simulink subsystem "rss_CurrCtlHybr"  (R2023a)
settings: Solver=VariableStepAuto  StartTime=0.0  StopTime=10.0  RelTol=1e-3
undefined symbols (not defined in the file): bit, Cdbl_indPhIndcMaxVal, Cdbl_indPhIndcPeakVal, Cdbl_iPhCurrMaxVal, Cdbl_iPhCurrPeakVal, Cdbl_nElecAgSpdMaxVal, Cdbl_nElecAgSpdPeakVal, Cdbl_psiPermMagFlxMaxVal, Cdbl_psiPermMagFlxPeakVal, Cdbl_uPhVltgMaxVal, Cdbl_uSplyVltgPeakVal, dt_Standardize_s16p15b0, ENM_MOTO_STATUS, Gbol_flgDaxQaxCurrClpFlg_C, Gu16_indDaxIndc_C, Gu16_indQaxIndc_C, Gu16_psiPermMagFlx_C
libraries: lib_conversion x18, lib_configurable_parameter x6, lib_discrete_time_PI_controller32bit x2, simulink x1
settings Model: Creator=CAV2OFO  LastModifiedBy=xiaoqiang.yuan
settings OptimizationCC: ReuseModelBlockBuffer=off

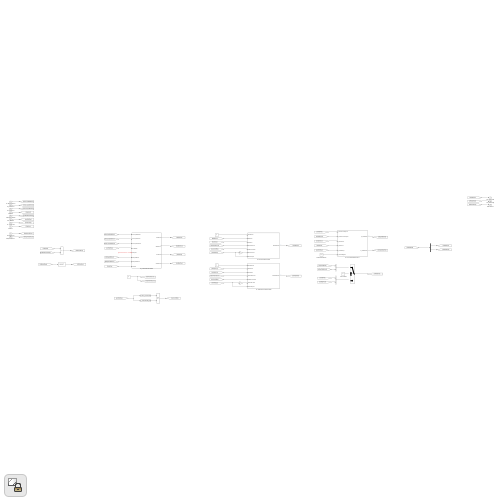
[thumbnail: Simulink's stored preview of the top-level diagram]
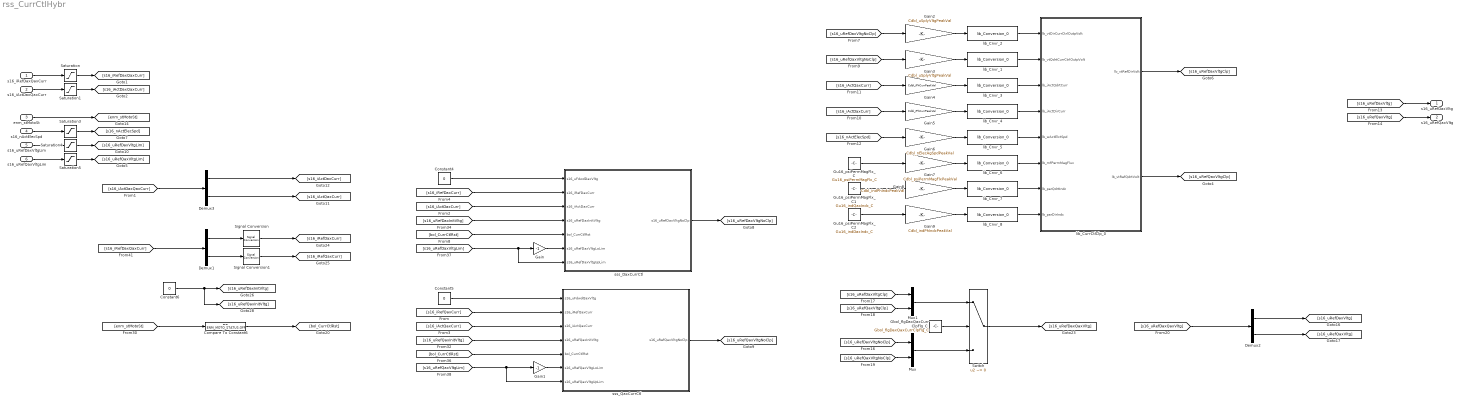
== system rss_CurrCtlHybr ==
  s16_iRefDaxQaxCurr : Inport  OutDataTypeStr=dt_Standardize_s16p15b0
  s16_iActDaxQaxCurr : Inport  Port=2  OutDataTypeStr=dt_Standardize_s16p15b0
  enm_stMotoSt : Inport  Port=3  OutDataTypeStr=Enum: ENM_MOTO_STATUS
  s16_nActElecSpd : Inport  Port=4  OutDataTypeStr=dt_Standardize_s16p15b0
  s16_uRefDaxVltgLim : Inport  Port=5  OutDataTypeStr=dt_Standardize_s16p15b0
  s16_uRefQaxVltgLim : Inport  Port=6  OutDataTypeStr=dt_Standardize_s16p15b0
  Compare To Constant6 : simulink/Logic and Bit Operations/Compare To Constant  relop===  const=ENM_MOTO_STATUS.OFF  OutDataTypeStr=boolean
  Constant4 : Constant  Value=0  OutDataTypeStr=dt_Standardize_s16p15b0
  Constant5 : Constant  Value=0  OutDataTypeStr=dt_Standardize_s16p15b0
  Constant6 : Constant  Value=0  OutDataTypeStr=dt_Standardize_s16p15b0
  Demux1 : Demux  Outputs=2
  Demux2 : Demux  Outputs=2
  Demux3 : Demux  Outputs=2
  Gain : Gain  Gain=-1  RndMeth=Simplest  OutDataTypeStr=Inherit: Same as input
  Gain1 : Gain  Gain=-1  RndMeth=Simplest  OutDataTypeStr=Inherit: Same as input
  Gain2 : Gain  Gain=Cdbl_uSplyVltgPeakVal  OutDataTypeStr=Inherit: Inherit via back propagation
  Gain3 : Gain  Gain=Cdbl_uSplyVltgPeakVal  OutDataTypeStr=Inherit: Inherit via back propagation
  Gain4 : Gain  Gain=Cdbl_iPhCurrPeakVal  OutDataTypeStr=Inherit: Inherit via back propagation
  Gain5 : Gain  Gain=Cdbl_iPhCurrPeakVal  OutDataTypeStr=Inherit: Inherit via back propagation
  Gain6 : Gain  Gain=Cdbl_nElecAgSpdPeakVal  OutDataTypeStr=Inherit: Inherit via back propagation
  Gain7 : Gain  Gain=Cdbl_psiPermMagFlxPeakVal  OutDataTypeStr=Inherit: Inherit via back propagation
  Gain8 : Gain  Gain=Cdbl_indPhIndcPeakVal  OutDataTypeStr=Inherit: Inherit via back propagation
  Gain9 : Gain  Gain=Cdbl_indPhIndcPeakVal  OutDataTypeStr=Inherit: Inherit via back propagation
  Gbol_flgDaxQaxCurrClpFlg_C : Constant  Value=Gbol_flgDaxQaxCurrClpFlg_C
  Gu16_psiPermMagFlx_C : Constant  Value=Gu16_psiPermMagFlx_C
  Gu16_psiPermMagFlx_C1 : Constant  Value=Gu16_indQaxIndc_C
  Gu16_psiPermMagFlx_C2 : Constant  Value=Gu16_indDaxIndc_C
  Mux : Mux  Inputs=2
  Mux1 : Mux  Inputs=2
  Saturation : Saturate  UpperLimit=Cdbl_iPhCurrMaxVal  LowerLimit=-Cdbl_iPhCurrMaxVal
  Saturation1 : Saturate  UpperLimit=Cdbl_iPhCurrMaxVal  LowerLimit=-Cdbl_iPhCurrMaxVal
  Saturation3 : Saturate  UpperLimit=Cdbl_nElecAgSpdMaxVal  LowerLimit=-Cdbl_nElecAgSpdMaxVal
  Saturation4 : Saturate  UpperLimit=Cdbl_uPhVltgMaxVal  LowerLimit=-Cdbl_uPhVltgMaxVal
  Saturation5 : Saturate  UpperLimit=Cdbl_uPhVltgMaxVal  LowerLimit=-Cdbl_uPhVltgMaxVal
  Signal Conversion : SignalConversion  OverrideOpt=off
  Signal Conversion1 : SignalConversion  OverrideOpt=off
  Switch : Switch  Criteria=u2 ~= 0  SaturateOnIntegerOverflow=off  InputSameDT=off
  lib_Cnvr_1 : lib_conversion/lib_Conversion_0  lb_parDataType=fixdt(1,16)  lb_parOutpMaxVal=Cdbl_uSplyVltgPeakVal  lb_parOutpMinVal=[]  RndMeth=Simplest  lb_parSatFlag=off
  lib_Cnvr_2 : lib_conversion/lib_Conversion_0  lb_parDataType=fixdt(1,16)  lb_parOutpMaxVal=Cdbl_uSplyVltgPeakVal  lb_parOutpMinVal=[]  RndMeth=Simplest  lb_parSatFlag=off
  lib_Cnvr_3 : lib_conversion/lib_Conversion_0  lb_parDataType=fixdt(1,16)  lb_parOutpMaxVal=Cdbl_iPhCurrPeakVal  lb_parOutpMinVal=[]  RndMeth=Simplest  lb_parSatFlag=off
  lib_Cnvr_4 : lib_conversion/lib_Conversion_0  lb_parDataType=fixdt(1,16)  lb_parOutpMaxVal=Cdbl_iPhCurrPeakVal  lb_parOutpMinVal=[]  RndMeth=Simplest  lb_parSatFlag=off
  lib_Cnvr_5 : lib_conversion/lib_Conversion_0  lb_parDataType=fixdt(1,16)  lb_parOutpMaxVal=Cdbl_nElecAgSpdPeakVal  lb_parOutpMinVal=[]  RndMeth=Simplest  lb_parSatFlag=off
  lib_Cnvr_6 : lib_conversion/lib_Conversion_0  lb_parDataType=fixdt(0,16)  lb_parOutpMaxVal=Cdbl_psiPermMagFlxPeakVal  lb_parOutpMinVal=[]  RndMeth=Simplest  lb_parSatFlag=off
  lib_Cnvr_7 : lib_conversion/lib_Conversion_0  lb_parDataType=fixdt(0,16)  lb_parOutpMaxVal=Cdbl_indPhIndcPeakVal  lb_parOutpMinVal=[]  RndMeth=Simplest  lb_parSatFlag=off
  lib_Cnvr_8 : lib_conversion/lib_Conversion_0  lb_parDataType=fixdt(0,16)  lb_parOutpMaxVal=Cdbl_indPhIndcPeakVal  lb_parOutpMinVal=[]  RndMeth=Simplest  lb_parSatFlag=off
  lib_CurrCtlClp_0 : Subsystem  mask{lb_parMaxPhsIndc=Cdbl_indPhIndcMaxVal*Cdbl_indPhIndcPeakVal, lb_parMaxElctSpd=Cdbl_nElecAgSpdMaxVal*Cdbl_nElecAgSpdPeakVal, lb_parMaxPhsCurr=Cdbl_iPhCurrMaxVal*Cdbl_iPhCurrPeakVal, lb_parMaxPermMagFlux=Cdbl_psiPermMagFlxMaxVal*Cdbl_psiPermMagFlxPeakVal, lb_parMaxCtrlPhsVolt=Cdbl_uPhVltgMaxVal*Cdbl_uSplyVltgPeakVal, lb_parOutpPekPhy=Cdbl_uSplyVltgPeakVal, lb_parOutpDataType=dt_Standardize_s16p15b0}
      mask prompts: lb_parMaxPhsIndc "Maximum phase inductance [H]:"; lb_parMaxElctSpd "Maximum electric speed [rad/s]:"; lb_parMaxPhsCurr "Maximum phase current [A]:"; lb_parMaxPermMagFlux "Maximum permanent magnet flux [Wb]:"; lb_parMaxCtrlPhsVolt "Maximum control phase voltage [V]:"; lb_parOutpPekPhy "Peak output physical value[V]:"; lb_parOutpDataType "Output data type:"
      mask init:
      | %% Define data type for operation w*L
      | lb_parOper1MaxVal = lb_parMaxElctSpd*lb_parMaxPhsIndc;
      | 
      | %% Define data type for operation w*L*I
      | lb_parOper2MaxVal = lb_parMaxElctSpd*lb_parMaxPhsIndc*lb_parMaxPhsCurr;
      | 
      | %% Define data type for operation w*PSI
      | lb_parOper3MaxVal = lb_parMaxElctSpd*lb_parMaxPermMagFlux;
      | 
      | %% Define data type for operation Vc+w*L*I
      | lb_parOper4MaxVal = lb_parMaxCtrlPhsVolt+lb_parMaxElctSpd*lb_parMaxPhsIndc*lb_parMaxPhsCurr;
      | 
      | %% Define data type for operation Vc+w*L*I+w*PSI
      | lb_parOper5MaxVal = lb_parOper4MaxVal+lb_parOper3MaxVal;
      mask DialogControl DescGroupVar Prompt: Current Coupling block
      mask DialogControl DescTextVar Prompt: This block computes the direct and quadrature voltage references.
      mask DialogControl modlPar Prompt: Parameters:
      mask DialogControl modlPar_copy Prompt: Data type:
  sss_DaxCurrCtl : Subsystem
  sss_QaxCurrCtl : Subsystem
  s16_uRefDaxVltg : Outport  OutDataTypeStr=dt_Standardize_s16p15b0
  s16_uRefQaxVltg : Outport  Port=2  OutDataTypeStr=dt_Standardize_s16p15b0
  wires:
  s16_iRefDaxQaxCurr/1 -> Saturation/1
  Demux2/2 -> [s16_uRefQaxVltg]
  [s16_uRefDaxQaxVltg] -> Demux2/1
  Gain/1 -> sss_DaxCurrCtl/6(s16_uRefDaxVltgLoLim)
  [s16_iActDaxQaxCurr] -> Demux3/1
  lib_Cnvr_8/1 -> lib_CurrCtlClp_0/8(lb_parDirIndc)
  Signal Conversion1/1 -> [s16_iRefQaxCurr]
  [s16_uRefDaxVltg] -> s16_uRefDaxVltg/1
  Gain7/1 -> lib_Cnvr_6/1
  Gu16_psiPermMagFlx_C2/1 -> Gain9/1
  Gain2/1 -> lib_Cnvr_2/1
  Gain6/1 -> lib_Cnvr_5/1
  lib_CurrCtlClp_0/1(lb_vtRefDirVolt) -> [s16_uRefDaxVltgClp]
  [s16_uRefDaxVltgNoClp] -> Mux/1
  Gu16_psiPermMagFlx_C1/1 -> Gain8/1
  Gbol_flgDaxQaxCurrClpFlg_C/1 -> Switch/2
  Gain8/1 -> lib_Cnvr_7/1
  Gu16_psiPermMagFlx_C/1 -> Gain7/1
  [s16_iActQaxCurr] -> Gain4/1
  [s16_nActElecSpd] -> Gain6/1
  Demux1/1 -> Signal Conversion/1
  Saturation5/1 -> [s16_uRefQaxVltgLim]
  [s16_uRefDaxVltgLim] -> Gain/1, sss_DaxCurrCtl/7(s16_uRefDaxVltgUpLim)
  sss_QaxCurrCtl/1(s16_uRefQaxVltgNoClp) -> [s16_uRefQaxVltgNoClp]
  [s16_uRefDaxVltgClp] -> Mux1/1
  [s16_uRefDaxVltgNoClp] -> Gain2/1
  Gain3/1 -> lib_Cnvr_1/1
  enm_stMotoSt/1 -> [enm_stMotoSt]
  Demux3/2 -> [s16_iActQaxCurr]
  [s16_iRefDaxQaxCurr] -> Demux1/1
  Signal Conversion/1 -> [s16_iRefDaxCurr]
  Saturation/1 -> [s16_iRefDaxQaxCurr]
  Saturation3/1 -> [s16_nActElecSpd]
  s16_uRefDaxVltgLim/1 -> Saturation4/1
  Demux2/1 -> [s16_uRefDaxVltg]
  lib_Cnvr_3/1 -> lib_CurrCtlClp_0/3(lb_iActQdrtCurr)
  Gain9/1 -> lib_Cnvr_8/1
  [s16_uRefQaxVltgLim] -> sss_QaxCurrCtl/7(s16_uRefQaxVltgUpLim), Gain1/1
  [bol_CurrCtlRst] -> sss_QaxCurrCtl/5(bol_CurrCtlRst)
  Demux1/2 -> Signal Conversion1/1
  Gain5/1 -> lib_Cnvr_4/1
  [s16_uRefQaxVltgNoClp] -> Gain3/1
  lib_Cnvr_7/1 -> lib_CurrCtlClp_0/7(lb_parQdrtIndc)
  s16_uRefQaxVltgLim/1 -> Saturation5/1
  Compare To Constant6/1 -> [bol_CurrCtlRst]
  Gain1/1 -> sss_QaxCurrCtl/6(s16_uRefQaxVltgLoLim)
  Saturation1/1 -> [s16_iActDaxQaxCurr]
  sss_DaxCurrCtl/1(s16_uRefDaxVltgNoClp) -> [s16_uRefDaxVltgNoClp]
  s16_nActElecSpd/1 -> Saturation3/1
  [s16_uRefDaxInitVltg] -> sss_DaxCurrCtl/4(s16_uRefDaxInitVltg)
  lib_CurrCtlClp_0/2(lb_vtRefQdrtVolt) -> [s16_uRefQaxVltgClp]
  lib_Cnvr_2/1 -> lib_CurrCtlClp_0/1(lb_vtDirCurrCtrlOutpVolt)
  [s16_uRefQaxVltg] -> s16_uRefQaxVltg/1
  lib_Cnvr_6/1 -> lib_CurrCtlClp_0/6(lb_mfPermMagFlux)
  [s16_uRefQaxVltgClp] -> Mux1/2
  Saturation4/1 -> [s16_uRefDaxVltgLim]
  [s16_iActDaxCurr] -> sss_DaxCurrCtl/3(s16_iActDaxCurr)
  Constant6/1 -> [s16_uRefDaxInitVltg], [s16_uRefQaxInitVltg]
  Constant4/1 -> sss_DaxCurrCtl/1(s16_uFdwdDaxVltg)
  [bol_CurrCtlRst] -> sss_DaxCurrCtl/5(bol_CurrCtlRst)
  [s16_uRefQaxVltgNoClp] -> Mux/2
  Mux/1 -> Switch/3
  [enm_stMotoSt] -> Compare To Constant6/1
  [s16_iRefQaxCurr] -> sss_QaxCurrCtl/2(s16_iRefQaxCurr)
  [s16_iActDaxCurr] -> Gain5/1
  [s16_iRefDaxCurr] -> sss_DaxCurrCtl/2(s16_iRefDaxCurr)
  Demux3/1 -> [s16_iActDaxCurr]
  s16_iActDaxQaxCurr/1 -> Saturation1/1
  Switch/1 -> [s16_uRefDaxQaxVltg]
  Gain4/1 -> lib_Cnvr_3/1
  lib_Cnvr_1/1 -> lib_CurrCtlClp_0/2(lb_vtQdrtCurrCtrlOutpVolt)
  Mux1/1 -> Switch/1
  [s16_iActQaxCurr] -> sss_QaxCurrCtl/3(s16_iActQaxCurr)
  Constant5/1 -> sss_QaxCurrCtl/1(s16_uFdwdQaxVltg)
  lib_Cnvr_5/1 -> lib_CurrCtlClp_0/5(lb_wActElctSpd)
  [s16_uRefQaxInitVltg] -> sss_QaxCurrCtl/4(s16_uRefQaxInitVltg)
  lib_Cnvr_4/1 -> lib_CurrCtlClp_0/4(lb_iActDirCurr)

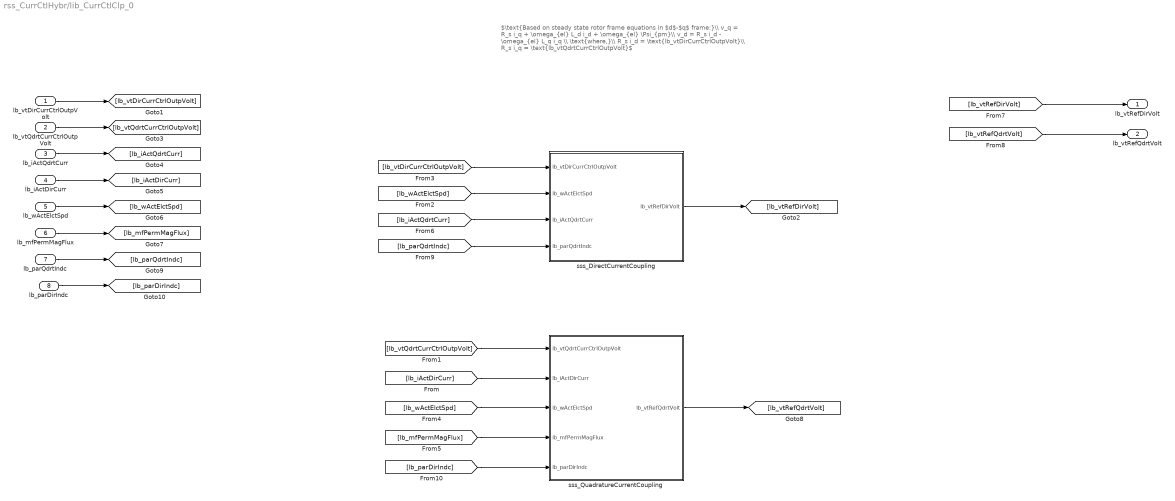
== system rss_CurrCtlHybr/lib_CurrCtlClp_0 ==
  note: $\text{Based on steady state rotor frame equations in $d$-$q$ frame:}\\ v_q = R_s i_q + \omega_{el} L_d i_d + \omega_{el} \Psi_{pm}\\ v_d = R_s i_d - \omega_{el} L_q i_q \\ \text{where,}\\ R_s i_d = \text{lb_vtDirCurrCtrlOutpVolt}\\ R_s i_q = \text{lb_vtQdrtCurrCtrlOutpVolt}$
  lb_vtDirCurrCtrlOutpVolt : Inport
  lb_vtQdrtCurrCtrlOutpVolt : Inport  Port=2
  lb_iActQdrtCurr : Inport  Port=3
  lb_iActDirCurr : Inport  Port=4
  lb_wActElctSpd : Inport  Port=5
  lb_mfPermMagFlux : Inport  Port=6
  lb_parQdrtIndc : Inport  Port=7
  lb_parDirIndc : Inport  Port=8
  sss_DirectCurrentCoupling : Subsystem
  sss_QuadratureCurrentCoupling : Subsystem
  lb_vtRefDirVolt : Outport
  lb_vtRefQdrtVolt : Outport  Port=2
  wires:
  [lb_parDirIndc] -> sss_QuadratureCurrentCoupling/5(lb_parDirIndc)
  lb_parDirIndc/1 -> [lb_parDirIndc]
  [lb_parQdrtIndc] -> sss_DirectCurrentCoupling/4(lb_parQdrtIndc)
  lb_parQdrtIndc/1 -> [lb_parQdrtIndc]
  [lb_iActDirCurr] -> sss_QuadratureCurrentCoupling/2(lb_iActDirCurr)
  [lb_vtQdrtCurrCtrlOutpVolt] -> sss_QuadratureCurrentCoupling/1(lb_vtQdrtCurrCtrlOutpVolt)
  lb_mfPermMagFlux/1 -> [lb_mfPermMagFlux]
  sss_DirectCurrentCoupling/1(lb_vtRefDirVolt) -> [lb_vtRefDirVolt]
  [lb_vtRefDirVolt] -> lb_vtRefDirVolt/1
  lb_wActElctSpd/1 -> [lb_wActElctSpd]
  [lb_iActQdrtCurr] -> sss_DirectCurrentCoupling/3(lb_iActQdrtCurr)
  [lb_mfPermMagFlux] -> sss_QuadratureCurrentCoupling/4(lb_mfPermMagFlux)
  lb_iActQdrtCurr/1 -> [lb_iActQdrtCurr]
  lb_vtQdrtCurrCtrlOutpVolt/1 -> [lb_vtQdrtCurrCtrlOutpVolt]
  sss_QuadratureCurrentCoupling/1(lb_vtRefQdrtVolt) -> [lb_vtRefQdrtVolt]
  [lb_wActElctSpd] -> sss_DirectCurrentCoupling/2(lb_wActElctSpd)
  [lb_vtRefQdrtVolt] -> lb_vtRefQdrtVolt/1
  lb_iActDirCurr/1 -> [lb_iActDirCurr]
  [lb_vtDirCurrCtrlOutpVolt] -> sss_DirectCurrentCoupling/1(lb_vtDirCurrCtrlOutpVolt)
  lb_vtDirCurrCtrlOutpVolt/1 -> [lb_vtDirCurrCtrlOutpVolt]
  [lb_wActElctSpd] -> sss_QuadratureCurrentCoupling/3(lb_wActElctSpd)

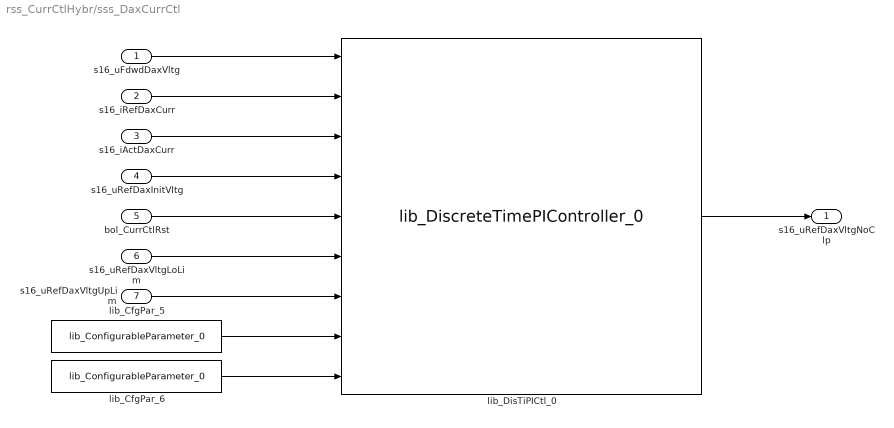
== system rss_CurrCtlHybr/sss_DaxCurrCtl ==
  s16_uFdwdDaxVltg : Inport
  s16_iRefDaxCurr : Inport  Port=2
  s16_iActDaxCurr : Inport  Port=3
  s16_uRefDaxInitVltg : Inport  Port=4
  bol_CurrCtlRst : Inport  Port=5
  s16_uRefDaxVltgLoLim : Inport  Port=6
  s16_uRefDaxVltgUpLim : Inport  Port=7
  lib_CfgPar_5 : lib_configurable_parameter/lib_ConfigurableParameter_0  lb_parCnfgPar=Gu16_facDaxCurrCtlKp_C  lb_parDataType=Inherit: Inherit from 'Constant value'  lb_parUpLim=Cdbl_facDaxCurrCtlKpMaxVal  lb_parLowLim=0
  lib_CfgPar_6 : lib_configurable_parameter/lib_ConfigurableParameter_0  lb_parCnfgPar=Gu16_facDaxCurrCtlKi_C  lb_parDataType=Inherit: Inherit from 'Constant value'  lb_parUpLim=Cdbl_facDaxCurrCtlKiMaxVal  lb_parLowLim=0
  lib_DisTiPICtl_0 : lib_discrete_time_PI_controller32bit/lib_DiscreteTimePIController_0  lb_parSampTime=Cdbl_tiMedTaskSmpTi  lb_parMaxSampTime=0.1  lb_parMaxPropGain=Cdbl_facDaxCurrCtlKpMaxVal  lb_parMaxIntgGain=Cdbl_facDaxCurrCtlKiMaxVal  lb_parRefInpMaxVal=Cdbl_iPhCurrMaxVal  lb_parRefInpMinVal=-Cdbl_iPhCurrMaxVal  lb_parMaxErrVal=2*Cdbl_iPhCurrMaxVal  lb_parMinErrVal=-2*Cdbl_iPhCurrMaxVal  lb_parMaxOutpVal=Cdbl_uPhVltgMaxVal  lb_parMinOutpVal=-Cdbl_uPhVltgMaxVal  lb_parAccmDataTypeMode=32-bit  lb_parOutpDataType=dt_Standardize_s16p15b0  lb_parSatMode=anti-windup with back-calculation
  s16_uRefDaxVltgNoClp : Outport
  wires:
  lib_CfgPar_5/1 -> lib_DisTiPICtl_0/8
  lib_CfgPar_6/1 -> lib_DisTiPICtl_0/9
  s16_uRefDaxVltgLoLim/1 -> lib_DisTiPICtl_0/6
  s16_iRefDaxCurr/1 -> lib_DisTiPICtl_0/2
  s16_iActDaxCurr/1 -> lib_DisTiPICtl_0/3
  s16_uFdwdDaxVltg/1 -> lib_DisTiPICtl_0/1
  lib_DisTiPICtl_0/1 -> s16_uRefDaxVltgNoClp/1
  s16_uRefDaxVltgUpLim/1 -> lib_DisTiPICtl_0/7
  s16_uRefDaxInitVltg/1 -> lib_DisTiPICtl_0/4
  bol_CurrCtlRst/1 -> lib_DisTiPICtl_0/5

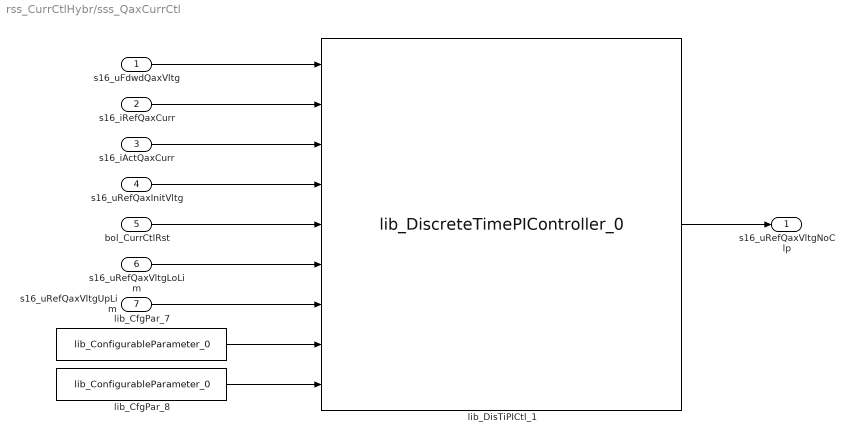
== system rss_CurrCtlHybr/sss_QaxCurrCtl ==
  s16_uFdwdQaxVltg : Inport
  s16_iRefQaxCurr : Inport  Port=2
  s16_iActQaxCurr : Inport  Port=3
  s16_uRefQaxInitVltg : Inport  Port=4
  bol_CurrCtlRst : Inport  Port=5
  s16_uRefQaxVltgLoLim : Inport  Port=6
  s16_uRefQaxVltgUpLim : Inport  Port=7
  lib_CfgPar_7 : lib_configurable_parameter/lib_ConfigurableParameter_0  lb_parCnfgPar=Gu16_facQaxCurrCtlKp_C  lb_parDataType=Inherit: Inherit from 'Constant value'  lb_parUpLim=Cdbl_facQaxCurrCtlKpMaxVal  lb_parLowLim=0
  lib_CfgPar_8 : lib_configurable_parameter/lib_ConfigurableParameter_0  lb_parCnfgPar=Gu16_facQaxCurrCtlKi_C  lb_parDataType=Inherit: Inherit from 'Constant value'  lb_parUpLim=Cdbl_facQaxCurrCtlKiMaxVal  lb_parLowLim=0
  lib_DisTiPICtl_1 : lib_discrete_time_PI_controller32bit/lib_DiscreteTimePIController_0  lb_parSampTime=Cdbl_tiMedTaskSmpTi  lb_parMaxSampTime=0.1  lb_parMaxPropGain=Cdbl_facQaxCurrCtlKpMaxVal  lb_parMaxIntgGain=Cdbl_facQaxCurrCtlKiMaxVal  lb_parRefInpMaxVal=Cdbl_iPhCurrMaxVal  lb_parRefInpMinVal=-Cdbl_iPhCurrMaxVal  lb_parMaxErrVal=2*Cdbl_iPhCurrMaxVal  lb_parMinErrVal=-2*Cdbl_iPhCurrMaxVal  lb_parMaxOutpVal=Cdbl_uPhVltgMaxVal  lb_parMinOutpVal=-Cdbl_uPhVltgMaxVal  lb_parAccmDataTypeMode=32-bit  lb_parOutpDataType=dt_Standardize_s16p15b0  lb_parSatMode=anti-windup with back-calculation
  s16_uRefQaxVltgNoClp : Outport
  wires:
  lib_CfgPar_7/1 -> lib_DisTiPICtl_1/8
  lib_CfgPar_8/1 -> lib_DisTiPICtl_1/9
  bol_CurrCtlRst/1 -> lib_DisTiPICtl_1/5
  s16_iRefQaxCurr/1 -> lib_DisTiPICtl_1/2
  s16_iActQaxCurr/1 -> lib_DisTiPICtl_1/3
  s16_uFdwdQaxVltg/1 -> lib_DisTiPICtl_1/1
  s16_uRefQaxInitVltg/1 -> lib_DisTiPICtl_1/4
  s16_uRefQaxVltgUpLim/1 -> lib_DisTiPICtl_1/7
  s16_uRefQaxVltgLoLim/1 -> lib_DisTiPICtl_1/6
  lib_DisTiPICtl_1/1 -> s16_uRefQaxVltgNoClp/1

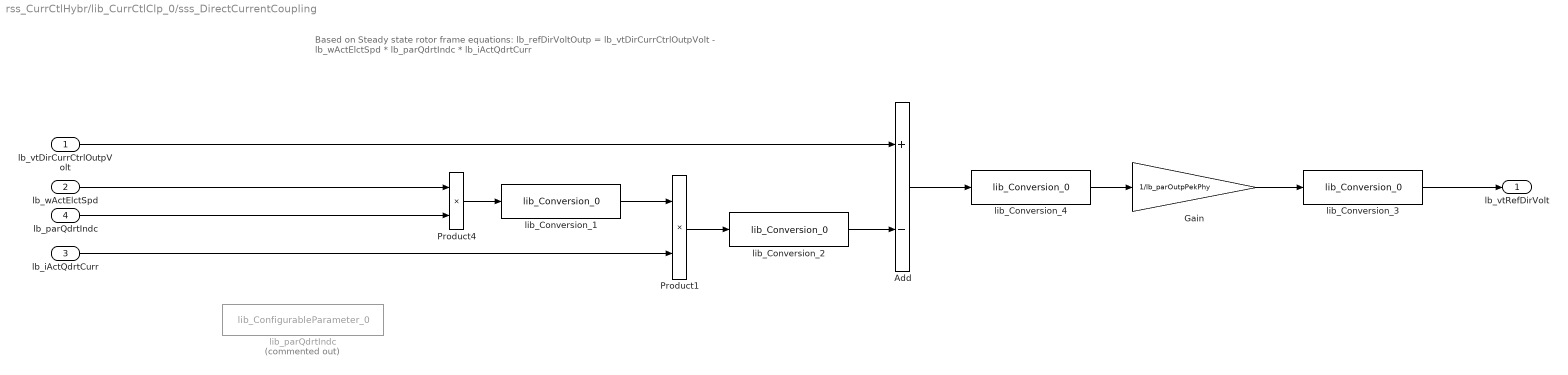
== system rss_CurrCtlHybr/lib_CurrCtlClp_0/sss_DirectCurrentCoupling ==
  note: Based on Steady state rotor frame equations:
      |
      | lb_refDirVoltOutp = lb_vtDirCurrCtrlOutpVolt
      | - lb_wActElctSpd * lb_parQdrtIndc * lb_iActQdrtCurr
  lb_vtDirCurrCtrlOutpVolt : Inport
  lb_wActElctSpd : Inport  Port=2
  lb_iActQdrtCurr : Inport  Port=3
  lb_parQdrtIndc : Inport  Port=4
  Add : Sum  Inputs=+-  OutDataTypeStr=Inherit: Inherit via back propagation
  Gain : Gain  Gain=1/lb_parOutpPekPhy  OutDataTypeStr=Inherit: Inherit via back propagation
  Product1 : Product  OutDataTypeStr=Inherit: Inherit via back propagation
  Product4 : Product  OutDataTypeStr=Inherit: Inherit via back propagation
  lib_Conversion_1 : lib_conversion/lib_Conversion_0  lb_parDataType=fixdt(1,16)  lb_parOutpMaxVal=lb_parOper1MaxVal  lb_parOutpMinVal=-lb_parOper1MaxVal  lb_parSatFlag=off
  lib_Conversion_2 : lib_conversion/lib_Conversion_0  lb_parDataType=fixdt(1,16)  lb_parOutpMaxVal=lb_parOper2MaxVal  lb_parOutpMinVal=-lb_parOper2MaxVal  lb_parSatFlag=off
  lib_Conversion_3 : lib_conversion/lib_Conversion_0  lb_parDataType=lb_parOutpDataType  lb_parOutpMaxVal=[]  lb_parOutpMinVal=[]  lb_parSatFlag=off
  lib_Conversion_4 : lib_conversion/lib_Conversion_0  lb_parDataType=fixdt(1,16)  lb_parOutpMaxVal=lb_parOper4MaxVal  lb_parOutpMinVal=-lb_parOper4MaxVal  lb_parSatFlag=off
  lib_parQdrtIndc : lib_configurable_parameter/lib_ConfigurableParameter_0  Commented=on  lb_parCnfgPar=lb_parQdrtIndc  lb_parDataType=Inherit: Inherit from 'Constant value'  lb_parUpLim=lb_parMaxPhsIndc  lb_parLowLim=0
  lb_vtRefDirVolt : Outport
  wires:
  lb_wActElctSpd/1 -> Product4/1
  lib_Conversion_2/1 -> Add/2
  lib_Conversion_1/1 -> Product1/1
  Product4/1 -> lib_Conversion_1/1
  lib_Conversion_3/1 -> lb_vtRefDirVolt/1
  Product1/1 -> lib_Conversion_2/1
  lb_iActQdrtCurr/1 -> Product1/2
  lb_vtDirCurrCtrlOutpVolt/1 -> Add/1
  lb_parQdrtIndc/1 -> Product4/2
  lib_Conversion_4/1 -> Gain/1
  Gain/1 -> lib_Conversion_3/1
  Add/1 -> lib_Conversion_4/1

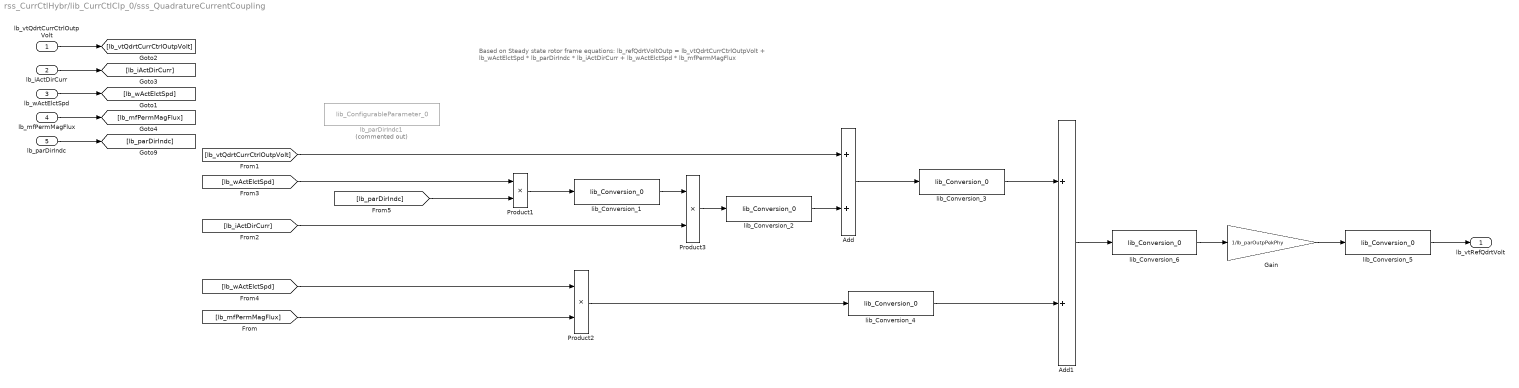
== system rss_CurrCtlHybr/lib_CurrCtlClp_0/sss_QuadratureCurrentCoupling ==
  note: Based on Steady state rotor frame equations:
      |
      | lb_refQdrtVoltOutp = lb_vtQdrtCurrCtrlOutpVolt +
      | lb_wActElctSpd * lb_parDirIndc * lb_iActDirCurr +
      | lb_wActElctSpd * lb_mfPermMagFlux
  lb_vtQdrtCurrCtrlOutpVolt : Inport
  lb_iActDirCurr : Inport  Port=2
  lb_wActElctSpd : Inport  Port=3
  lb_mfPermMagFlux : Inport  Port=4
  lb_parDirIndc : Inport  Port=5
  Add : Sum  OutDataTypeStr=Inherit: Inherit via back propagation
  Add1 : Sum  OutDataTypeStr=Inherit: Inherit via back propagation
  Gain : Gain  Gain=1/lb_parOutpPekPhy  OutDataTypeStr=Inherit: Inherit via back propagation
  Product1 : Product  OutDataTypeStr=Inherit: Inherit via back propagation
  Product2 : Product  OutDataTypeStr=Inherit: Inherit via back propagation
  Product3 : Product  OutDataTypeStr=Inherit: Inherit via back propagation
  lb_parDirIndc1 : lib_configurable_parameter/lib_ConfigurableParameter_0  Commented=on  lb_parCnfgPar=lb_parDirIndc  lb_parDataType=Inherit: Inherit from 'Constant value'  lb_parUpLim=lb_parMaxPhsIndc  lb_parLowLim=0
  lib_Conversion_1 : lib_conversion/lib_Conversion_0  lb_parDataType=fixdt(1,16)  lb_parOutpMaxVal=lb_parOper1MaxVal  lb_parOutpMinVal=-lb_parOper1MaxVal  lb_parSatFlag=off
  lib_Conversion_2 : lib_conversion/lib_Conversion_0  lb_parDataType=fixdt(1,16)  lb_parOutpMaxVal=lb_parOper2MaxVal  lb_parOutpMinVal=-lb_parOper2MaxVal  lb_parSatFlag=off
  lib_Conversion_3 : lib_conversion/lib_Conversion_0  lb_parDataType=fixdt(1,16)  lb_parOutpMaxVal=lb_parOper4MaxVal  lb_parOutpMinVal=-lb_parOper4MaxVal  lb_parSatFlag=off
  lib_Conversion_4 : lib_conversion/lib_Conversion_0  lb_parDataType=fixdt(1,16)  lb_parOutpMaxVal=lb_parOper3MaxVal  lb_parOutpMinVal=-lb_parOper3MaxVal  lb_parSatFlag=off
  lib_Conversion_5 : lib_conversion/lib_Conversion_0  lb_parDataType=lb_parOutpDataType  lb_parOutpMaxVal=[]  lb_parOutpMinVal=[]  lb_parSatFlag=off
  lib_Conversion_6 : lib_conversion/lib_Conversion_0  lb_parDataType=fixdt(1,16)  lb_parOutpMaxVal=lb_parOper5MaxVal  lb_parOutpMinVal=-lb_parOper5MaxVal  lb_parSatFlag=off
  lb_vtRefQdrtVolt : Outport
  wires:
  lb_parDirIndc/1 -> [lb_parDirIndc]
  lib_Conversion_4/1 -> Add1/2
  Product2/1 -> lib_Conversion_4/1
  lib_Conversion_3/1 -> Add1/1
  Add/1 -> lib_Conversion_3/1
  lib_Conversion_2/1 -> Add/2
  Product3/1 -> lib_Conversion_2/1
  lib_Conversion_1/1 -> Product3/1
  [lb_wActElctSpd] -> Product1/1
  [lb_iActDirCurr] -> Product3/2
  Product1/1 -> lib_Conversion_1/1
  [lb_parDirIndc] -> Product1/2
  [lb_vtQdrtCurrCtrlOutpVolt] -> Add/1
  [lb_wActElctSpd] -> Product2/1
  [lb_mfPermMagFlux] -> Product2/2
  lib_Conversion_5/1 -> lb_vtRefQdrtVolt/1
  lb_mfPermMagFlux/1 -> [lb_mfPermMagFlux]
  lb_wActElctSpd/1 -> [lb_wActElctSpd]
  lb_iActDirCurr/1 -> [lb_iActDirCurr]
  lb_vtQdrtCurrCtrlOutpVolt/1 -> [lb_vtQdrtCurrCtrlOutpVolt]
  lib_Conversion_6/1 -> Gain/1
  Add1/1 -> lib_Conversion_6/1
  Gain/1 -> lib_Conversion_5/1
